simulink model "PID_controlinput_tracking_delay"  (R2022a)
settings: Solver=VariableStepAuto  StartTime=0.0  StopTime=10.0  RelTol=1e-3
libraries: cstblocks x4
settings Model: Creator=Linxi Ren  LastModifiedBy=Linxi Ren

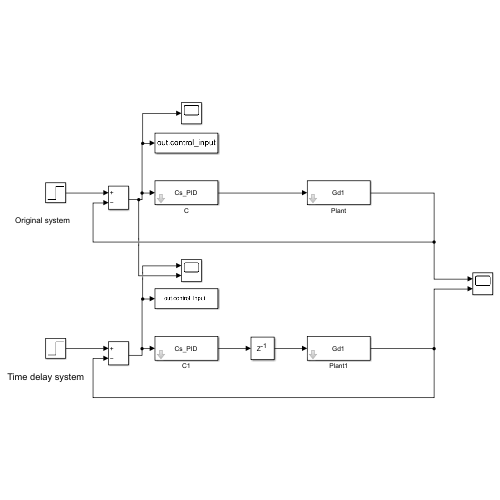
[thumbnail: Simulink's stored preview of the top-level diagram]
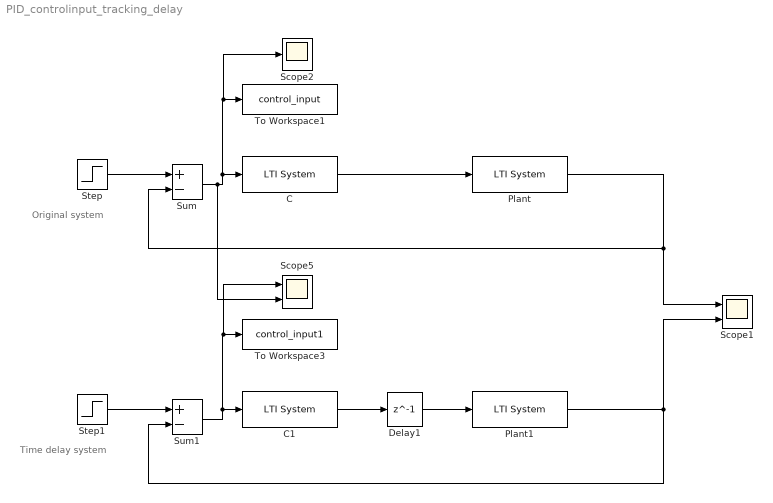
== system PID_controlinput_tracking_delay ==
  note: Time delay system
  note: Original system
  C : cstblocks/LTI System  sys=Cs_PID  IC=[]
  C1 : cstblocks/LTI System  sys=Cs_PID  IC=[]
  Delay1 : Delay  DelayLength=1  InitialCondition=0
  Plant : cstblocks/LTI System  sys=Gd1  IC=[]
  Plant1 : cstblocks/LTI System  sys=Gd1  IC=[]
  Scope1 : Scope  NumInputPorts=2
  Scope2 : Scope
  Scope5 : Scope  NumInputPorts=2
  Step : Step  Time=0  SampleTime=0.0325
  Step1 : Step  Time=0  SampleTime=0.0325
  Sum : Sum  Inputs=+-  InputSameDT=on  SaturateOnIntegerOverflow=on  OutDataTypeStr=Inherit: Same as first input
  Sum1 : Sum  Inputs=+-  InputSameDT=on  SaturateOnIntegerOverflow=on  OutDataTypeStr=Inherit: Same as first input
  To Workspace1 : ToWorkspace  VariableName=control_input  SaveFormat=Timeseries  SampleTime=-1
  To Workspace3 : ToWorkspace  VariableName=control_input1  SaveFormat=Timeseries  SampleTime=-1
  wires:
  Plant/1 -> Scope1/1, Sum/2
  Sum/1 -> Scope2/1, To Workspace1/1, C/1, Scope5/2
  C/1 -> Plant/1
  Step/1 -> Sum/1
  Step1/1 -> Sum1/1
  Sum1/1 -> Scope5/1, To Workspace3/1, C1/1
  Plant1/1 -> Scope1/2, Sum1/2
  C1/1 -> Delay1/1
  Delay1/1 -> Plant1/1
